simulink model "hil3_target_demo"  (Simulink 7.3)
settings: Solver=ode3  SolverMode=SingleTasking  StartTime=0.0  StopTime=10.0  RelTol=1e-3
PreLoadFcn:
  | waijung.modelPreload; % Required for working with Waijung Blockset. Do not remove.
undefined symbols (not defined in the file): HSEOSC, Link, LQFP176, ST, STM32F417IG
libraries: stm32f4_device_config_lib x1
CloseFcn:
  | waijung.modelClose; % Required for working with Waijung Blockset. Do not remove.
settings Model: Creator=Krisada  LastModifiedBy=Krisada
settings OptimizationCC: OptimizeModelRefInitCode=on  LifeSpan=1
settings HardwareCC: ProdEndianess=LittleEndian  ProdHWDeviceType=ARM Compatible->Cortex - M4  TargetEndianess=LittleEndian  TargetHWDeviceType=ARM Compatible->Cortex - M4
settings RTWCC: SystemTargetFile=stm32f4.tlc  GenerateMakefile=off  TemplateMakefile=ert_default_tmf  Description=STM32F4 Target  ProcessScript=stm32f4_make_rtw_hook
settings CodeAppCC: IgnoreCustomStorageClasses=off
settings STFCustomTargetCC: ModelReferenceCompliant=off  CombineOutputUpdateFcns=on  ERTCustomFileBanners=on  SupportContinuousTime=off  SupportNonInlinedSFcns=off  SystemTargetFile=stm32f4.tlc
settings ERTTargetCC: MultiwordLength=2048  ModelReferenceCompliant=off  ParMdlRefBuildCompliant=off  CompOptLevelCompliant=off  ERTFirstTimeCompliant=off  ModelStepFunctionPrototypeControlCompliant=off  CPPClassGenCompliant=off  InlinedParameterPlacement=NonHierarchical  ERTSrcFileBannerTemplate=stm32f4_code_template.cgt  ERTHdrFileBannerTemplate=stm32f4_code_template.cgt  ERTDataSrcFileTemplate=stm32f4_code_template.cgt  ERTDataHdrFileTemplate=stm32f4_code_template.cgt  ERTCustomFileTemplate=stm32f4_file_process.tlc

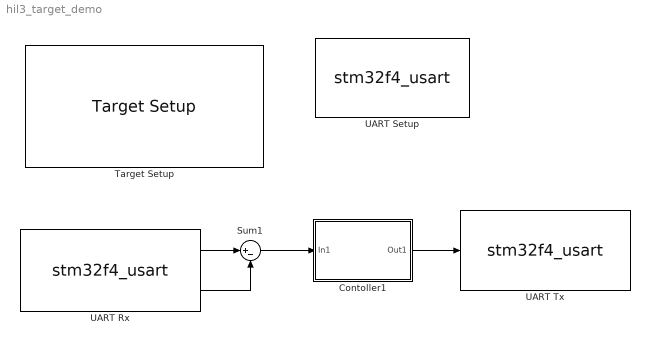
== system hil3_target_demo ==
  Contoller1 : Subsystem
  Sum1 : Sum  Inputs=|+-  OutDataType=fixdt(1, 16)  OutScaling=2^0
  Target Setup : stm32f4_device_config_lib/Target Setup  Priority=100  compiler=GNU ARM  previous_compiler=GNU ARM  mcu=STM32F417IG (LQFP176)  mcustr=STM32F417IG  clockconfig=HSEOSC-8MHz  system_stm32f4xx_c_path=F:\trunk\targets\stm32f4_target\stm32f4\utils\system_stm32f4xx_default\STM32F40_41xxx\hseosc8mhz  showmemoryconfiguration=off  stacksize=0x2000  heapsize=0x2000  enableautocompiledownload=on  fullchiperase=off  programmerinterface=ST-Link  editctrlstr=on  compilercontrolstr=$(patsubst %, -I%, .) -mcpu=cortex-m4 -mthumb -mthumb-interwork -mfloat-abi=hard -mfpu=fpv4-sp-d16 -ffast-math -Wall -Wextra -Ofast  assemblercontrolstr=$(patsubst %, -I%, .) -mcpu=cortex-m4 -mthumb -mthumb-interwork -mfloat-abi=hard -mfpu=fpv4-sp-d16 -ffast-math -Wall -Wextra -Ofast -Wa,-amhls=$(<:.s=.lst) -D__STACK_SIZE=$(STACK_SIZE) -D__HEAP_SIZE=$(HEAP_SIZE)  linkercontrolstr=-T$(LD_SCRIPT) -g -Wl,-Map=$(MAP),--cref,--no-warn-mismatch -mcpu=cortex-m4 -mthumb -mthumb-interwork -mfloat-abi=hard -mfpu=fpv4-sp-d16 -specs=nosys.specs  runafterdownload=on  execprofile=None  profileruart=3  profilerbaud=500000  profilertxpin=D8  profilerinitstr=0.001,168000000,168000,500000,0  manualsetsampletime=off  sampletime=0.001  blockid=TargetSetup  systickreloadvalue=168000  hseval=8000000  lastprofileruart=3  hclk=168000000  flashorigin=0x8000000  flashlength=1024k  ramorigin=0x20000000  ramlength=128k  useextram=off
  UART Rx : S-Function  Priority=1  FunctionName=stm32f4_usart  Parameters=configuration,uartmodule,transfer,baudrate,inputtype,outputtype,confstr,binheaderarray,binterminatorarray,asciiheader,asciiterminator,bindatalength,packetmode,varname,sampletime,sampletimestr,blockid  EnableBusSupport=off  mask(stm32f4_usart){configuration=Rx, uartmodule=3, baudrate=115200, databits=8, parity=No, stopbit=1, remaptxpin=Not used, remaprxpin=Not used, flowcontrol=None, remapctspin=Not used, remaprtspin=Not used, advanceoptions=off, rxbuffersize=512, txbuffersize=512, transfer=Blocking, packetmode=Binary, binheader='7E 7E', binterminator='03 03', porttype_double=2, porttype_single=0, porttype_int8=0, porttype_uint8=0, porttype_int16=0, porttype_uint16=0, porttype_int32=0, porttype_uint32=0, asciiformat='value=%d,%f', rx_asciiterminator=CRLF (0x0D 0x0A - "\r\n"), tx_asciiterminator=LF (0x0A - "\n"), storagename=<empty>, varname=, inputtype=[0], outputtype=[2  0 0], binheaderarray=[2 126  126], binterminatorarray=[2 3  3], bindatalength=16, asciiheader='value=%d,%f\r\n', asciiterminator=[2 13 10], sampletime=.005, sampletimestr=0.005, blockid=UARTRx, confstr=[ "dummy", "0", "*", "*", "0", "*", "*", "0", "*", "*", "0", "*", "*", "1", "4", "3", "1", "4", "1", "512", "512", "1", "3", "115200", "8", "No", "1", "None", "USART3"], lastmodule=1}
      mask prompts: uartmodule "UART Module"; baudrate "Baud rate (bps)"; databits "Data bits"; stopbit "Stop bit"; remaptxpin "Tx Pin"; remaprxpin "Rx Pin"; flowcontrol "Hardware flow control"; remapctspin "HW Flow control, CTS Pin"; remaprtspin "HW Flow control, RTS Pin"; advanceoptions "Advance options"; rxbuffersize "Rx buffer size (bytes)"; txbuffersize "Tx buffer size (bytes)"; packetmode "Packet mode"; binheader "Binary header (example: '7E 7E')"; binterminator "Binary terminator (example: '03 03')"; porttype_double "Number of data port, type DOUBLE"; porttype_single "Number of data port, type SINGLE"; porttype_int8 "Number of data port, type INT8"; porttype_uint8 "Number of data port, type UINT8"; porttype_int16 "Number of data port, type INT16"; porttype_uint16 "Number of data port, type UINT16"; porttype_int32 "Number of data port, type INT32"; porttype_uint32 "Number of data port, type UINT32"; asciiformat "Ascii format"; rx_asciiterminator "End of packet"; tx_asciiterminator "End of packet"; storagename "Buffer"; varname "Var name"; inputtype "Input data type"; outputtype "Output data type"; binheaderarray "Binary header"; binterminatorarray "Binary terminator"; bindatalength "Binary data length"; asciiheader "Ascii header (printf format)"; asciiterminator "Ascii terminator"; sampletime "Sample time (sec)"; sampletimestr "Compiled sample time (sec) in string"; confstr "Configuration string"; lastmodule "Last module selected"
      mask help:
      | Data type for Ascii format
      | %u, %i, %d, %o, %x: uint32
      | %e, %g, %f: single
      | %c: int8
      mask init:
      | stm32f4_usart_callback('init');
      mask Help: web(fullfile(waijungdocroot,'stm32f4_usart_rx.htm'), '-browser')
      mask StyleString: popup(Setup|Tx|Rx),popup(1|2|3|4|5|6),edit,popup(8),popup(No|Odd|Even),popup(0.5|1|1.5|2),popup(Not used|A9|B6),popup(Not used|A10|B7),popup(None|RTS|CTS|RTS/CTS),popup(Not used|A11),popup(Not used|A12),checkbox,popup(16|32|64|128|256|512|1024|2048),popup(16|32|64|128|256|512|1024|2048),popup(Blocking|Non-Blocking),popup(Ascii|Binary|String Buffer),edit,edit,edit,edit,edit,edit,edit,edit,edit,edit,edit,popup(CR (0x0D - "\r")|LF (0x0A - "\n")|CRLF (0x0D 0x0A - "\r\n")),popup(CR (0x0D - "\r")|LF (0x0A - "\n")|CRLF (0x0D 0x0A - "\r\n")|None),popup(<empty>),edit,edit,edit,edit,edit,edit,edit,edit,edit,edit,edit,edit,edit
      mask CallbackString: stm32f4_usart_callback('configuration');|stm32f4_usart_callback('uartmodule');|stm32f4_usart_callback('baudrate');||||||stm32f4_usart_callback('flowcontrol');|||stm32f4_usart_callback('advanceoptions');|||stm32f4_usart_callback('transfer');|stm32f4_usart_callback('packetmode');|stm32f4_usart_callback('binheader');|stm32f4_usart_callback('binterminator');|stm32f4_usart_callback('porttype');|stm32f4_usart_callback('porttype');|stm32f4_usart_callback('porttype');|stm32f4_usart_callback('porttype');|stm32f4_usart_callback('porttype');|stm32f4_usart_callback('porttype');|stm32f4_usart_callback('porttype');|stm32f4_usart_callback('porttype');|stm32f4_usart_callback('asciiformat');|stm32f4_usart_callback('rx_asciiterminator');|stm32f4_usart_callback('tx_asciiterminator');|stm32f4_usart_callback('storagename');|stm32f4_usart_callback('varname');||||||||stm32f4_usart_callback('sampletime');|stm32f4_usart_callback('sampletimestr');|stm32f4_usart_callback('blockid');||
      mask Display: text(0.05, 0.5, 'Module: USART3_Rx\nPacket: Binary\nTransfer: Blocking\nTs (sec): 0.005','ver','middle','hor','left'); port_label('output', 1,'double'); port_label('output', 2,'double');
  UART Setup : S-Function  Priority=1  FunctionName=stm32f4_usart  Parameters=configuration,uartmodule,transfer,baudrate,inputtype,outputtype,confstr,binheaderarray,binterminatorarray,asciiheader,asciiterminator,bindatalength,packetmode,varname,sampletime,sampletimestr,blockid  EnableBusSupport=off  mask(stm32f4_usart){configuration=Setup, uartmodule=3, baudrate=115200, databits=8, parity=No, stopbit=1, remaptxpin=D8, remaprxpin=D9, flowcontrol=None, remapctspin=Not used, remaprtspin=Not used, advanceoptions=off, rxbuffersize=512, txbuffersize=512, transfer=Blocking, packetmode=Ascii, binheader='7E 7E', binterminator='03 03', porttype_double=1, porttype_single=0, porttype_int8=1, porttype_uint8=0, porttype_int16=0, porttype_uint16=0, porttype_int32=0, porttype_uint32=0, asciiformat='%d,%f', rx_asciiterminator=CRLF (0x0D 0x0A - "\r\n"), tx_asciiterminator=CR (0x0D - "\r"), storagename=<empty>, varname=, inputtype=[0], outputtype=[0], binheaderarray=[0], binterminatorarray=[0], bindatalength=0, asciiheader='', asciiterminator=[0], sampletime=-1, sampletimestr=0.005, blockid=UARTSetup, confstr=[ "dummy", "1", "D", "8", "1", "D", "9", "0", "*", "*", "0", "*", "*", "1", "4", "3", "1", "4", "1", "512", "512", "1", "3", "115200", "8", "No", "1", "None", "USART3"], lastmodule=3}
      mask prompts: uartmodule "UART Module"; baudrate "Baud rate (bps)"; databits "Data bits"; stopbit "Stop bit"; remaptxpin "Tx Pin"; remaprxpin "Rx Pin"; flowcontrol "Hardware flow control"; remapctspin "HW Flow control, CTS Pin"; remaprtspin "HW Flow control, RTS Pin"; advanceoptions "Advance options"; rxbuffersize "Rx buffer size (bytes)"; txbuffersize "Tx buffer size (bytes)"; packetmode "Packet mode"; binheader "Binary header (example: '7E 7E')"; binterminator "Binary terminator (example: '03 03')"; porttype_double "Number of data port, type DOUBLE"; porttype_single "Number of data port, type SINGLE"; porttype_int8 "Number of data port, type INT8"; porttype_uint8 "Number of data port, type UINT8"; porttype_int16 "Number of data port, type INT16"; porttype_uint16 "Number of data port, type UINT16"; porttype_int32 "Number of data port, type INT32"; porttype_uint32 "Number of data port, type UINT32"; asciiformat "Ascii format"; rx_asciiterminator "End of packet"; tx_asciiterminator "End of packet"; storagename "Buffer"; varname "Var name"; inputtype "Input data type"; outputtype "Output data type"; binheaderarray "Binary header"; binterminatorarray "Binary terminator"; bindatalength "Binary data length"; asciiheader "Ascii header (printf format)"; asciiterminator "Ascii terminator"; sampletime "Sample time (sec)"; sampletimestr "Compiled sample time (sec) in string"; confstr "Configuration string"; lastmodule "Last module selected"
      mask help:
      | Default STM32F4DISCOVERY + aMG F4 Connect 2 + aMG USB Converter N2 settings use
      |
      | USART3, Tx D8, Rx D9 and USB Serial Converter A.
      mask init:
      | stm32f4_usart_callback('init');
      mask Help: web(fullfile(waijungdocroot,'stm32f4_usart_setup.htm'), '-browser')
      mask StyleString: popup(Setup|Tx|Rx),popup(1|2|3|4|5|6),edit,popup(8),popup(No|Odd|Even),popup(0.5|1|1.5|2),popup(Not used|B10|C10|D8),popup(Not used|B11|C11|D9),popup(None|RTS|CTS|RTS/CTS),popup(Not used|B13|D11),popup(Not used|B14|D12),checkbox,popup(16|32|64|128|256|512|1024|2048),popup(16|32|64|128|256|512|1024|2048),popup(Blocking|Non-Blocking),popup(Ascii|Binary|String Buffer),edit,edit,edit,edit,edit,edit,edit,edit,edit,edit,edit,popup(CR (0x0D - "\r")|LF (0x0A - "\n")|CRLF (0x0D 0x0A - "\r\n")),popup(CR (0x0D - "\r")|LF (0x0A - "\n")|CRLF (0x0D 0x0A - "\r\n")|None),popup(<empty>),edit,edit,edit,edit,edit,edit,edit,edit,edit,edit,edit,edit,edit
      mask CallbackString: stm32f4_usart_callback('configuration');|stm32f4_usart_callback('uartmodule');|stm32f4_usart_callback('baudrate');||||||stm32f4_usart_callback('flowcontrol');|||stm32f4_usart_callback('advanceoptions');|||stm32f4_usart_callback('transfer');|stm32f4_usart_callback('packetmode');|stm32f4_usart_callback('binheader');|stm32f4_usart_callback('binterminator');|stm32f4_usart_callback('porttype');|stm32f4_usart_callback('porttype');|stm32f4_usart_callback('porttype');|stm32f4_usart_callback('porttype');|stm32f4_usart_callback('porttype');|stm32f4_usart_callback('porttype');|stm32f4_usart_callback('porttype');|stm32f4_usart_callback('porttype');|stm32f4_usart_callback('asciiformat');|stm32f4_usart_callback('rx_asciiterminator');|stm32f4_usart_callback('tx_asciiterminator');|stm32f4_usart_callback('storagename');|stm32f4_usart_callback('varname');||||||||stm32f4_usart_callback('sampletime');|stm32f4_usart_callback('sampletimestr');|stm32f4_usart_callback('blockid');||
      mask Display: text(0.5, 0.5, 'Module: USART3_Setup\nBaud (Bps): 115200\nDMA Buffer: 512/512\nTx/Rx Pin: D8/D9','ver','middle','hor','center');
  UART Tx : S-Function  Priority=1  FunctionName=stm32f4_usart  Parameters=configuration,uartmodule,transfer,baudrate,inputtype,outputtype,confstr,binheaderarray,binterminatorarray,asciiheader,asciiterminator,bindatalength,packetmode,varname,sampletime,sampletimestr,blockid  EnableBusSupport=off  mask(stm32f4_usart){configuration=Tx, uartmodule=3, baudrate=115200, databits=8, parity=No, stopbit=1, remaptxpin=Not used, remaprxpin=Not used, flowcontrol=None, remapctspin=Not used, remaprtspin=Not used, advanceoptions=off, rxbuffersize=512, txbuffersize=512, transfer=Blocking, packetmode=Binary, binheader='7E 7E', binterminator='03 03', porttype_double=1, porttype_single=0, porttype_int8=0, porttype_uint8=0, porttype_int16=0, porttype_uint16=0, porttype_int32=0, porttype_uint32=0, asciiformat='value=%d,%f', rx_asciiterminator=CRLF (0x0D 0x0A - "\r\n"), tx_asciiterminator=CRLF (0x0D 0x0A - "\r\n"), storagename=<empty>, varname=, inputtype=[1  0], outputtype=[0], binheaderarray=[2 126  126], binterminatorarray=[2 3  3], bindatalength=8, asciiheader='value=%d,%f\r\n', asciiterminator=[2 13 10], sampletime=0.005, sampletimestr=0.005, blockid=UARTTx, confstr=[ "dummy", "0", "*", "*", "0", "*", "*", "0", "*", "*", "0", "*", "*", "1", "4", "3", "1", "4", "1", "512", "512", "1", "3", "115200", "8", "No", "1", "None", "USART3"], lastmodule=1}
      mask prompts: uartmodule "UART Module"; baudrate "Baud rate (bps)"; databits "Data bits"; stopbit "Stop bit"; remaptxpin "Tx Pin"; remaprxpin "Rx Pin"; flowcontrol "Hardware flow control"; remapctspin "HW Flow control, CTS Pin"; remaprtspin "HW Flow control, RTS Pin"; advanceoptions "Advance options"; rxbuffersize "Rx buffer size (bytes)"; txbuffersize "Tx buffer size (bytes)"; packetmode "Packet mode"; binheader "Binary header (example: '7E 7E')"; binterminator "Binary terminator (example: '03 03')"; porttype_double "Number of data port, type DOUBLE"; porttype_single "Number of data port, type SINGLE"; porttype_int8 "Number of data port, type INT8"; porttype_uint8 "Number of data port, type UINT8"; porttype_int16 "Number of data port, type INT16"; porttype_uint16 "Number of data port, type UINT16"; porttype_int32 "Number of data port, type INT32"; porttype_uint32 "Number of data port, type UINT32"; asciiformat "Ascii format"; rx_asciiterminator "End of packet"; tx_asciiterminator "End of packet"; storagename "Buffer"; varname "Var name"; inputtype "Input data type"; outputtype "Output data type"; binheaderarray "Binary header"; binterminatorarray "Binary terminator"; bindatalength "Binary data length"; asciiheader "Ascii header (printf format)"; asciiterminator "Ascii terminator"; sampletime "Sample time (sec)"; sampletimestr "Compiled sample time (sec) in string"; confstr "Configuration string"; lastmodule "Last module selected"
      mask help:
      | Data type for Ascii format
      | %u, %i, %d, %o, %x: uint32
      | %e, %g, %f: single
      | %c: int8
      mask init:
      | stm32f4_usart_callback('init');
      mask Help: web(fullfile(waijungdocroot,'stm32f4_usart_tx.htm'), '-browser')
      mask StyleString: popup(Setup|Tx|Rx),popup(1|2|3|4|5|6),edit,popup(8),popup(No|Odd|Even),popup(0.5|1|1.5|2),popup(Not used|A9|B6),popup(Not used|A10|B7),popup(None|RTS|CTS|RTS/CTS),popup(Not used|A11),popup(Not used|A12),checkbox,popup(16|32|64|128|256|512|1024|2048),popup(16|32|64|128|256|512|1024|2048),popup(Blocking|Non-Blocking),popup(Ascii|Binary|String Buffer),edit,edit,edit,edit,edit,edit,edit,edit,edit,edit,edit,popup(CR (0x0D - "\r")|LF (0x0A - "\n")|CRLF (0x0D 0x0A - "\r\n")),popup(CR (0x0D - "\r")|LF (0x0A - "\n")|CRLF (0x0D 0x0A - "\r\n")|None),popup(<empty>),edit,edit,edit,edit,edit,edit,edit,edit,edit,edit,edit,edit,edit
      mask CallbackString: stm32f4_usart_callback('configuration');|stm32f4_usart_callback('uartmodule');|stm32f4_usart_callback('baudrate');||||||stm32f4_usart_callback('flowcontrol');|||stm32f4_usart_callback('advanceoptions');|||stm32f4_usart_callback('transfer');|stm32f4_usart_callback('packetmode');|stm32f4_usart_callback('binheader');|stm32f4_usart_callback('binterminator');|stm32f4_usart_callback('porttype');|stm32f4_usart_callback('porttype');|stm32f4_usart_callback('porttype');|stm32f4_usart_callback('porttype');|stm32f4_usart_callback('porttype');|stm32f4_usart_callback('porttype');|stm32f4_usart_callback('porttype');|stm32f4_usart_callback('porttype');|stm32f4_usart_callback('asciiformat');|stm32f4_usart_callback('rx_asciiterminator');|stm32f4_usart_callback('tx_asciiterminator');|stm32f4_usart_callback('storagename');|stm32f4_usart_callback('varname');||||||||stm32f4_usart_callback('sampletime');|stm32f4_usart_callback('sampletimestr');|stm32f4_usart_callback('blockid');||
      mask Display: text(0.95, 0.5, 'Module: USART3_Tx\nPacket: Binary\nTransfer: Blocking\nTs (sec): 0.005','ver','middle','hor','right'); port_label('input', 1,'double');
  wires:
  Contoller1/1(Out1) -> UART Tx/1
  UART Rx/1 -> Sum1/1
  Sum1/1 -> Contoller1/1(In1)
  UART Rx/2 -> Sum1/2

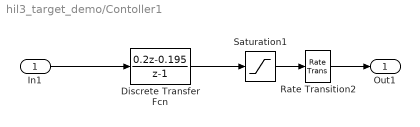
== system hil3_target_demo/Contoller1 ==
  In1 : Inport
  Discrete Transfer Fcn : DiscreteTransferFcn  Numerator=[0.2 -0.195]  Denominator=[1 -1]  SampleTime=-1
  Rate Transition2 : RateTransition
  Saturation1 : Saturate  UpperLimit=100  LowerLimit=-100  LinearizeAsGain=off  ZeroCross=off  OutDataType=fixdt(1, 16)  OutScaling=2^0
  Out1 : Outport
  wires:
  Rate Transition2/1 -> Out1/1
  Discrete Transfer Fcn/1 -> Saturation1/1
  In1/1 -> Discrete Transfer Fcn/1
  Saturation1/1 -> Rate Transition2/1
